simulink model "main_pipeline"  (R2021a)
settings: Solver=FixedStepDiscrete  StartTime=0.0  StopTime=0  RelTol=1e-3
undefined symbols (not defined in the file): gray, Rec, SDTV, strel
libraries: visiontextngfix x9, visionmorphops x7, visionstatistics x3, visionconversions x2, visionsources x1
settings Model: Creator=leonardoaraujo  LastModifiedBy=leonardoaraujo

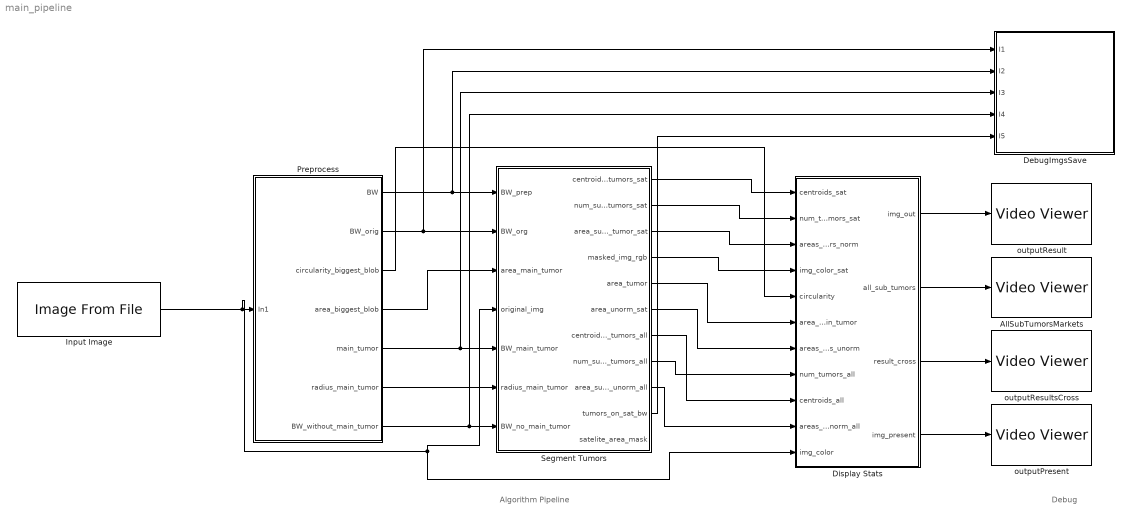
== system main_pipeline ==
  note: Algorithm Pipeline
  note: Debug
  AllSubTumorsMarkets : VideoViewer  colormapValue=gray(256)  FigPos=[659 848 678 632]
  DebugImgsSave : MATLAB Function  TreatAsAtomicUnit=on
  Display Stats : Subsystem
  Input Image : visionsources/Image From File  Tag=vipblks_nd  FileName=/Users/leonardoaraujo/Desktop/Cher Experiment/C6R_OV_BiggerBrain.jpg  Ts=inf  imagePorts=One multidimensional signal  OutPortLabels=R|G|B  ImageDataType=Inherit from input image  sdImageDataType=uint(8)  Signed=on  WordLength=16  FractionLengthMode=User-defined  FractionLength=15
  Preprocess : Subsystem  mask{open_1=8, erode_1=2, close_1=10}
      mask prompts: open_1 "Open Blobs"; erode_1 "Pre-clean"; close_1 "Close Main tumor"
  Segment Tumors : Subsystem  mask{erode_1=2, sat_area=150}
      mask prompts: erode_1 "Filter Small Artifacts"; sat_area "Satelite Area"
  outputPresent : VideoViewer  colormapValue=gray(256)  FigPos=[1 849 1440 721]
  outputResult : VideoViewer  colormapValue=gray(256)  FigPos=[180 848 678 632]
  outputResultsCross : VideoViewer  colormapValue=gray(256)  FigPos=[415 815 678 632]
  wires:
  Input Image/1 -> Segment Tumors/4(original_img), Display Stats/11(img_color), Preprocess/1(In1)
  Preprocess/1(BW) -> DebugImgsSave/2(I2), Segment Tumors/1(BW_prep)
  Preprocess/2(BW_orig) -> DebugImgsSave/1(I1), Segment Tumors/2(BW_org)
  Segment Tumors/1(centroid_sub_tumors_sat) -> Display Stats/1(centroids_sat)
  Segment Tumors/2(num_sub_tumors_sat) -> Display Stats/2(num_tumors_sat)
  Segment Tumors/3(area_sub_tumor_sat) -> Display Stats/3(areas_sub_tumors_norm)
  Preprocess/3(circularity_biggest_blob) -> Display Stats/5(circularity)
  Preprocess/4(area_biggest_blob) -> Segment Tumors/3(area_main_tumor)
  Segment Tumors/4(masked_img_rgb) -> Display Stats/4(img_color_sat)
  Segment Tumors/5(area_tumor) -> Display Stats/6(area_main_tumor)
  Segment Tumors/10(tumors_on_sat_bw) -> DebugImgsSave/5(I5)
  Segment Tumors/6(area_unorm_sat) -> Display Stats/7(areas_sub_tumors_unorm)
  Display Stats/1(img_out) -> outputResult/1
  Segment Tumors/8(num_sub_tumors_all) -> Display Stats/8(num_tumors_all)
  Segment Tumors/7(centroid_sub_tumors_all) -> Display Stats/9(centroids_all)
  Segment Tumors/9(area_sub_tumors_unorm_all) -> Display Stats/10(areas_sub_tumors_unorm_all)
  Display Stats/2(all_sub_tumors) -> AllSubTumorsMarkets/1
  Preprocess/5(main_tumor) -> DebugImgsSave/3(I3), Segment Tumors/5(BW_main_tumor)
  Preprocess/6(radius_main_tumor) -> Segment Tumors/6(radius_main_tumor)
  Preprocess/7(BW_without_main_tumor) -> DebugImgsSave/4(I4), Segment Tumors/7(BW_no_main_tumor)
  Display Stats/3(result_cross) -> outputResultsCross/1
  Display Stats/4(img_present) -> outputPresent/1

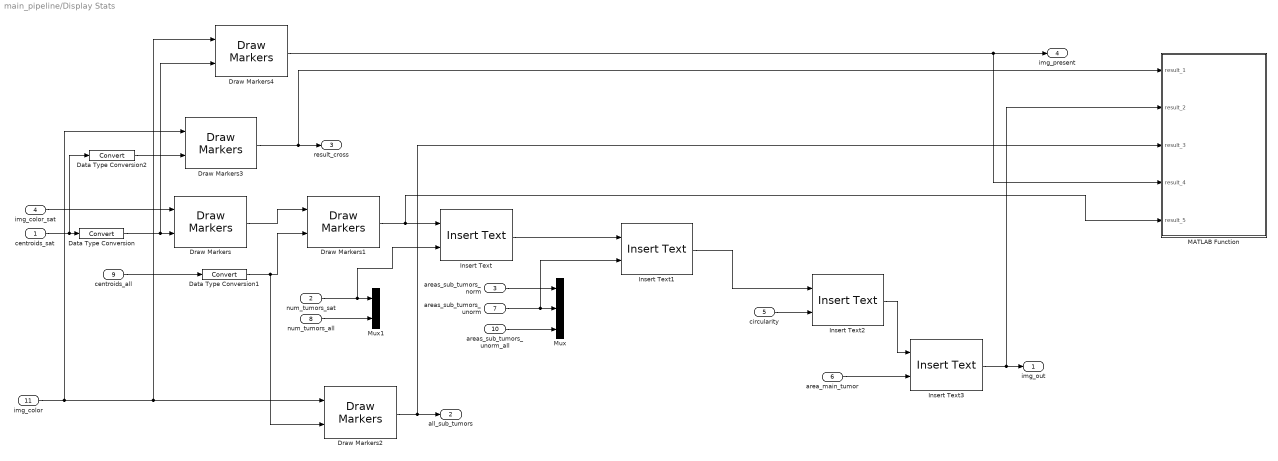
== system main_pipeline/Display Stats ==
  centroids_sat : Inport
  num_tumors_sat : Inport  Port=2
  areas_sub_tumors_norm : Inport  Port=3
  img_color_sat : Inport  Port=4
  circularity : Inport  Port=5
  area_main_tumor : Inport  Port=6
  areas_sub_tumors_unorm : Inport  Port=7
  num_tumors_all : Inport  Port=8
  centroids_all : Inport  Port=9
  areas_sub_tumors_unorm_all : Inport  Port=10
  img_color : Inport  Port=11
  Data Type Conversion : DataTypeConversion
  Data Type Conversion1 : DataTypeConversion
  Data Type Conversion2 : DataTypeConversion
  Draw Markers : visiontextngfix/Draw Markers  shape=Circle  size=30  fill=on  fillClrSource=Specify via dialog  display=User-specified value  intensity=200  color=[200 0 0]  opacity=0.6  viewport=Entire image  antialiasing=off  inType=Obsolete  imagePorts=One multidimensional signal  roundingMode=Floor  overflowMode=off  memoryMode=Specify word length  memoryWordLength=16  memoryFracLength=15  prodOutputMode=Binary point scaling  prodOutputWordLength=32  prodOutputFracLength=14
      settings: SourceProductBaseCode=VP
  Draw Markers1 : visiontextngfix/Draw Markers  shape=Circle  size=10  fill=on  fillClrSource=Specify via dialog  display=User-specified value  intensity=200  color=[0 0 200]  opacity=0.3  viewport=Entire image  antialiasing=off  inType=Obsolete  imagePorts=One multidimensional signal  roundingMode=Floor  overflowMode=off  memoryMode=Specify word length  memoryWordLength=16  memoryFracLength=15  prodOutputMode=Binary point scaling  prodOutputWordLength=32  prodOutputFracLength=14
      settings: SourceProductBaseCode=VP
  Draw Markers2 : visiontextngfix/Draw Markers  shape=Circle  size=10  fill=on  fillClrSource=Specify via dialog  display=User-specified value  intensity=200  color=[0 0 200]  opacity=0.3  viewport=Entire image  antialiasing=off  inType=Obsolete  imagePorts=One multidimensional signal  roundingMode=Floor  overflowMode=off  memoryMode=Specify word length  memoryWordLength=16  memoryFracLength=15  prodOutputMode=Binary point scaling  prodOutputWordLength=32  prodOutputFracLength=14
      settings: SourceProductBaseCode=VP
  Draw Markers3 : visiontextngfix/Draw Markers  shape=Plus  size=30  fill=on  fillClrSource=Specify via dialog  display=User-specified value  intensity=200  color=[200 0 0]  opacity=0.6  viewport=Entire image  antialiasing=off  inType=Obsolete  imagePorts=One multidimensional signal  roundingMode=Floor  overflowMode=off  memoryMode=Specify word length  memoryWordLength=16  memoryFracLength=15  prodOutputMode=Binary point scaling  prodOutputWordLength=32  prodOutputFracLength=14
      settings: SourceProductBaseCode=VP
  Draw Markers4 : visiontextngfix/Draw Markers  shape=Circle  size=30  fill=on  fillClrSource=Specify via dialog  display=User-specified value  intensity=200  color=[200 0 0]  opacity=0.6  viewport=Entire image  antialiasing=off  inType=Obsolete  imagePorts=One multidimensional signal  roundingMode=Floor  overflowMode=off  memoryMode=Specify word length  memoryWordLength=16  memoryFracLength=15  prodOutputMode=Binary point scaling  prodOutputWordLength=32  prodOutputFracLength=14
      settings: SourceProductBaseCode=VP
  Insert Text : visiontextngfix/Insert Text  inputType=Obsolete  theText='#Satellite Lesion: %2d'  getTextLocFrom=Specify via dialog  textLoc=[1 1]  getTextColorFrom=Specify via dialog  textColor=[0 255 0]  getTextIntensityFrom=Specify via dialog  textIntensity=100  getTextOpacityFrom=Specify via dialog  textOpacity=1.0  dummyVar2=0  dummyVar3=0  dummyVar4=0  imagePorts=One multidimensional signal  isInputTransposed=off  fontFace=LucidaSansRegular  dummyVar1=0  blockFontSize=25  antiAliased=on
      settings: SourceProductBaseCode=VP
  Insert Text1 : visiontextngfix/Insert Text  inputType=Obsolete  theText='Satellite Lesion Total Area: %2f'  getTextLocFrom=Specify via dialog  textLoc=[1 50]  getTextColorFrom=Specify via dialog  textColor=[0 255 0]  getTextIntensityFrom=Specify via dialog  textIntensity=100  getTextOpacityFrom=Specify via dialog  textOpacity=1.0  dummyVar2=0  dummyVar3=0  dummyVar4=0  imagePorts=One multidimensional signal  isInputTransposed=off  fontFace=LucidaSansRegular  dummyVar1=0  blockFontSize=25  antiAliased=on
      settings: SourceProductBaseCode=VP
  Insert Text2 : visiontextngfix/Insert Text  inputType=Obsolete  theText='Surface Irregularity: %2f'  getTextLocFrom=Specify via dialog  textLoc=[1 100]  getTextColorFrom=Specify via dialog  textColor=[0 255 0]  getTextIntensityFrom=Specify via dialog  textIntensity=100  getTextOpacityFrom=Specify via dialog  textOpacity=1.0  dummyVar2=0  dummyVar3=0  dummyVar4=0  imagePorts=One multidimensional signal  isInputTransposed=off  fontFace=LucidaSansRegular  dummyVar1=0  blockFontSize=25  antiAliased=on
      settings: SourceProductBaseCode=VP
  Insert Text3 : visiontextngfix/Insert Text  inputType=Obsolete  theText='Main tumor Size: %d'  getTextLocFrom=Specify via dialog  textLoc=[1 150]  getTextColorFrom=Specify via dialog  textColor=[0 255 0]  getTextIntensityFrom=Specify via dialog  textIntensity=100  getTextOpacityFrom=Specify via dialog  textOpacity=1.0  dummyVar2=0  dummyVar3=0  dummyVar4=0  imagePorts=One multidimensional signal  isInputTransposed=off  fontFace=LucidaSansRegular  dummyVar1=0  blockFontSize=25  antiAliased=on
      settings: SourceProductBaseCode=VP
  MATLAB Function : MATLAB Function  TreatAsAtomicUnit=on
  Mux : Mux  Inputs=3
  Mux1 : Mux  Inputs=2
  img_out : Outport
  all_sub_tumors : Outport  Port=2
  result_cross : Outport  Port=3
  img_present : Outport  Port=4
  wires:
  Data Type Conversion/1 -> Draw Markers4/2, Draw Markers/2
  centroids_sat/1 -> Data Type Conversion2/1, Data Type Conversion/1
  img_color_sat/1 -> Draw Markers/1
  Insert Text/1 -> Insert Text1/1
  Insert Text1/1 -> Insert Text2/1
  circularity/1 -> Insert Text2/2
  Insert Text2/1 -> Insert Text3/1
  Insert Text3/1 -> MATLAB Function/2(result_2), img_out/1
  area_main_tumor/1 -> Insert Text3/2
  areas_sub_tumors_norm/1 -> Mux/1
  areas_sub_tumors_unorm/1 -> Insert Text1/2, Mux/2
  num_tumors_sat/1 -> Insert Text/2, Mux1/1
  Draw Markers/1 -> Draw Markers1/1
  Draw Markers1/1 -> MATLAB Function/5(result_5), Insert Text/1
  centroids_all/1 -> Data Type Conversion1/1
  Data Type Conversion1/1 -> Draw Markers2/2, Draw Markers1/2
  areas_sub_tumors_unorm_all/1 -> Mux/3
  Draw Markers2/1 -> MATLAB Function/3(result_3), all_sub_tumors/1
  img_color/1 -> Draw Markers2/1, Draw Markers4/1, Draw Markers3/1
  Data Type Conversion2/1 -> Draw Markers3/2
  Draw Markers3/1 -> MATLAB Function/1(result_1), result_cross/1
  Draw Markers4/1 -> img_present/1, MATLAB Function/4(result_4)
  num_tumors_all/1 -> Mux1/2

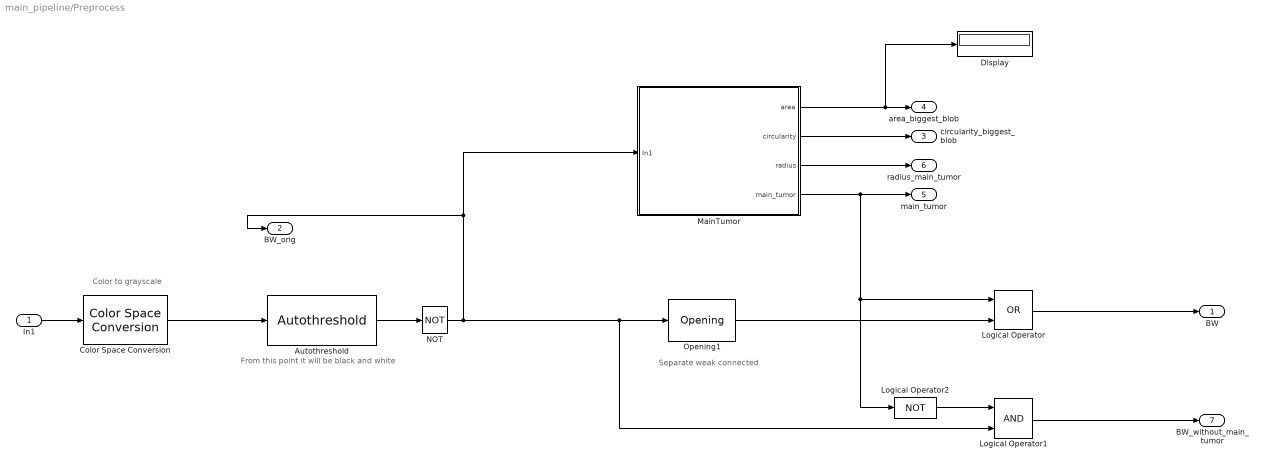
== system main_pipeline/Preprocess ==
  note: From this point it will be black and white
  note: Color to grayscale
  note: Separate weak connected
  In1 : Inport
  Autothreshold : visionconversions/Autothreshold  operator=>  threshOut=off  effMetricOut=off  userDefinedRange=off  umin=0  umax=255  outOfRngOpt=Ignore  scaleThreshold=off  scaleFactor=1  roundingMode=Floor  overflowMode=off  P1Mode=Specify word length  P1WordLength=32  P1FracLength=30  P2Mode=Specify word length  P2WordLength=32  P2FracLength=22  P3Mode=Specify word length  P3WordLength=32  P3FracLength=14  P4Mode=Binary point scaling  P4WordLength=32  P4FracLength=15  Q1Mode=Specify word length  Q1WordLength=32  Q1FracLength=16  EMMode=Specify word length  EMWordLength=16  EMFracLength=14
      settings: SourceProductBaseCode=VP
  Color Space Conversion : visionconversions/Color Space  Conversion  conversion=Obsolete  conversionActive=R'G'B' to intensity  wp_str=D65  rec=Rec. 601 (SDTV)  sys=1125/60/2:1  imagePorts=One multidimensional signal
  Display : Display
  Logical Operator : Logic  Operator=OR  AllPortsSameDT=off  OutDataTypeStr=boolean
  Logical Operator1 : Logic  AllPortsSameDT=off  OutDataTypeStr=boolean
  Logical Operator2 : Logic  Operator=NOT  AllPortsSameDT=off  OutDataTypeStr=boolean
  MainTumor : Subsystem
  NOT : Logic  Operator=NOT  IconShape=distinctive  AllPortsSameDT=off  OutDataTypeStr=boolean
  Opening1 : visionmorphops/Opening  nhoodsrc=Specify via dialog  strel=strel('disk',open_1)
      settings: SourceProductBaseCode=VP
  BW : Outport
  BW_orig : Outport  Port=2
  circularity_biggest_blob : Outport  Port=3
  area_biggest_blob : Outport  Port=4
  main_tumor : Outport  Port=5
  radius_main_tumor : Outport  Port=6
  BW_without_main_tumor : Outport  Port=7
  wires:
  Autothreshold/1 -> NOT/1
  In1/1 -> Color Space Conversion/1
  Opening1/1 -> Logical Operator/2
  Color Space Conversion/1 -> Autothreshold/1
  MainTumor/2(circularity) -> circularity_biggest_blob/1
  MainTumor/3(radius) -> radius_main_tumor/1
  MainTumor/4(main_tumor) -> Logical Operator2/1, Logical Operator/1, main_tumor/1
  MainTumor/1(area) -> Display/1, area_biggest_blob/1
  Logical Operator/1 -> BW/1
  Logical Operator2/1 -> Logical Operator1/1
  Logical Operator1/1 -> BW_without_main_tumor/1
  NOT/1 -> Logical Operator1/2, Opening1/1, MainTumor/1(In1), BW_orig/1

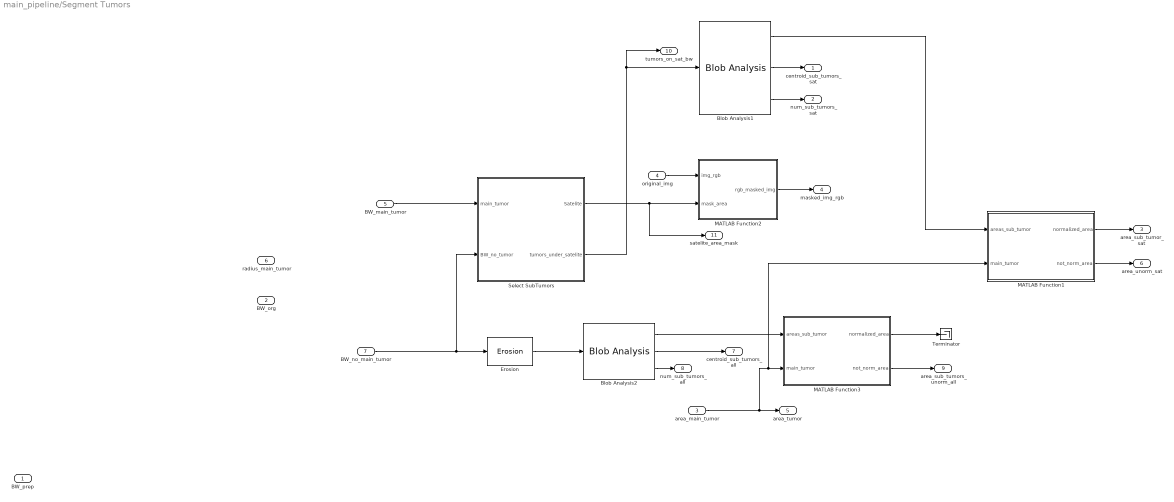
== system main_pipeline/Segment Tumors ==
  BW_prep : Inport
  BW_org : Inport  Port=2
  area_main_tumor : Inport  Port=3
  original_img : Inport  Port=4
  BW_main_tumor : Inport  Port=5
  radius_main_tumor : Inport  Port=6
  BW_no_main_tumor : Inport  Port=7
  Blob Analysis1 : visionstatistics/Blob Analysis  Tag=vipblks_row_conv  area=on  centroid=on  bBox=off  majorAxis=off  minorAxis=off  angle=off  eccentricity=off  equivDiameterSq=off  extent=off  perimeter=off  outDT=double  conn=8  isLabel=off  maxBlobs=500  warnIfNumBlobsExceeded=on  isCount=on  useMinArea=off  minArea=0  useMaxArea=off  maxArea=intmax('uint32')  excludeBorderBlob=on  isOutVarDim=off  isFill=on  fillValues=-1  roundingMode=Floor  overflowMode=off  prodOutputMode=Binary point scaling  prodOutputWordLength=32  prodOutputFracLength=16  accumMode=Binary point scaling  accumWordLength=32  accumFracLength=0  outputMode=Binary point scaling  outputWordLength=32  outputFracLength=16  firstCoeffMode=Binary point scaling  firstCoeffWordLength=16  firstCoeffFracLength=14  secondCoeffMode=Binary point scaling  secondCoeffWordLength=32  secondCoeffFracLength=16
  Blob Analysis2 : visionstatistics/Blob Analysis  Tag=vipblks_row_conv  area=on  centroid=on  bBox=off  majorAxis=off  minorAxis=off  angle=off  eccentricity=off  equivDiameterSq=off  extent=off  perimeter=off  outDT=double  conn=8  isLabel=off  maxBlobs=500  warnIfNumBlobsExceeded=on  isCount=on  useMinArea=off  minArea=0  useMaxArea=off  maxArea=intmax('uint32')  excludeBorderBlob=on  isOutVarDim=off  isFill=on  fillValues=-1  roundingMode=Floor  overflowMode=off  prodOutputMode=Binary point scaling  prodOutputWordLength=32  prodOutputFracLength=16  accumMode=Binary point scaling  accumWordLength=32  accumFracLength=0  outputMode=Binary point scaling  outputWordLength=32  outputFracLength=16  firstCoeffMode=Binary point scaling  firstCoeffWordLength=16  firstCoeffFracLength=14  secondCoeffMode=Binary point scaling  secondCoeffWordLength=32  secondCoeffFracLength=16
  Erosion : visionmorphops/Erosion  nhoodsrc=Specify via dialog  strel=strel('disk',erode_1)
      settings: SourceProductBaseCode=VP
  MATLAB Function1 : MATLAB Function  TreatAsAtomicUnit=on
  MATLAB Function2 : MATLAB Function  TreatAsAtomicUnit=on
  MATLAB Function3 : MATLAB Function  TreatAsAtomicUnit=on
  Select SubTumors : Subsystem
  Terminator : Terminator
  centroid_sub_tumors_sat : Outport
  num_sub_tumors_sat : Outport  Port=2
  area_sub_tumor_sat : Outport  Port=3
  masked_img_rgb : Outport  Port=4
  area_tumor : Outport  Port=5
  area_unorm_sat : Outport  Port=6
  centroid_sub_tumors_all : Outport  Port=7
  num_sub_tumors_all : Outport  Port=8
  area_sub_tumors_unorm_all : Outport  Port=9
  tumors_on_sat_bw : Outport  Port=10
  satelite_area_mask : Outport  Port=11
  wires:
  Blob Analysis2/2 -> centroid_sub_tumors_all/1
  Blob Analysis2/1 -> MATLAB Function3/1(areas_sub_tumor)
  Blob Analysis2/3 -> num_sub_tumors_all/1
  MATLAB Function3/1(normalized_area) -> Terminator/1
  MATLAB Function3/2(not_norm_area) -> area_sub_tumors_unorm_all/1
  area_main_tumor/1 -> MATLAB Function1/2(main_tumor), MATLAB Function3/2(main_tumor), area_tumor/1
  BW_no_main_tumor/1 -> Select SubTumors/2(BW_no_tumor), Erosion/1
  BW_main_tumor/1 -> Select SubTumors/1(main_tumor)
  MATLAB Function2/1(rgb_masked_img) -> masked_img_rgb/1
  original_img/1 -> MATLAB Function2/1(img_rgb)
  Select SubTumors/1(Satelite) -> satelite_area_mask/1, MATLAB Function2/2(mask_area)
  Select SubTumors/2(tumors_under_satelite) -> tumors_on_sat_bw/1, Blob Analysis1/1
  Blob Analysis1/1 -> MATLAB Function1/1(areas_sub_tumor)
  Blob Analysis1/2 -> centroid_sub_tumors_sat/1
  Blob Analysis1/3 -> num_sub_tumors_sat/1
  MATLAB Function1/2(not_norm_area) -> area_unorm_sat/1
  MATLAB Function1/1(normalized_area) -> area_sub_tumor_sat/1
  Erosion/1 -> Blob Analysis2/1

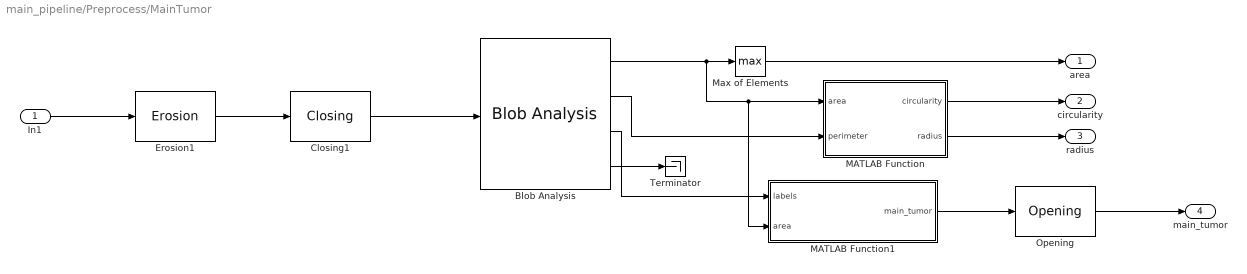
== system main_pipeline/Preprocess/MainTumor ==
  In1 : Inport
  Blob Analysis : visionstatistics/Blob Analysis  Tag=vipblks_row_conv  area=on  centroid=off  bBox=off  majorAxis=off  minorAxis=off  angle=off  eccentricity=off  equivDiameterSq=off  extent=off  perimeter=on  outDT=double  conn=8  isLabel=on  maxBlobs=50  warnIfNumBlobsExceeded=on  isCount=on  useMinArea=on  minArea=200  useMaxArea=off  maxArea=intmax('uint32')  excludeBorderBlob=on  isOutVarDim=off  isFill=on  fillValues=-1  roundingMode=Floor  overflowMode=off  prodOutputMode=Binary point scaling  prodOutputWordLength=32  prodOutputFracLength=16  accumMode=Binary point scaling  accumWordLength=32  accumFracLength=0  outputMode=Binary point scaling  outputWordLength=32  outputFracLength=16  firstCoeffMode=Binary point scaling  firstCoeffWordLength=16  firstCoeffFracLength=14  secondCoeffMode=Binary point scaling  secondCoeffWordLength=32  secondCoeffFracLength=16
  Closing1 : visionmorphops/Closing  nhoodsrc=Specify via dialog  strel=strel('disk',close_1)
      settings: SourceProductBaseCode=VP
  Erosion1 : visionmorphops/Erosion  nhoodsrc=Specify via dialog  strel=strel('disk',erode_1)
      settings: SourceProductBaseCode=VP
  MATLAB Function : MATLAB Function  TreatAsAtomicUnit=on
  MATLAB Function1 : MATLAB Function  TreatAsAtomicUnit=on
  Max of Elements : MinMax  Function=max
  Opening : visionmorphops/Opening  nhoodsrc=Specify via dialog  strel=strel('disk',30)
      settings: SourceProductBaseCode=VP
  Terminator : Terminator
  area : Outport
  circularity : Outport  Port=2
  radius : Outport  Port=3
  main_tumor : Outport  Port=4
  wires:
  Blob Analysis/4 -> Terminator/1
  In1/1 -> Erosion1/1
  Blob Analysis/3 -> MATLAB Function1/1(labels)
  Max of Elements/1 -> area/1
  Blob Analysis/1 -> MATLAB Function/1(area), MATLAB Function1/2(area), Max of Elements/1
  MATLAB Function/2(radius) -> radius/1
  MATLAB Function/1(circularity) -> circularity/1
  Blob Analysis/2 -> MATLAB Function/2(perimeter)
  Erosion1/1 -> Closing1/1
  Closing1/1 -> Blob Analysis/1
  Opening/1 -> main_tumor/1
  MATLAB Function1/1(main_tumor) -> Opening/1

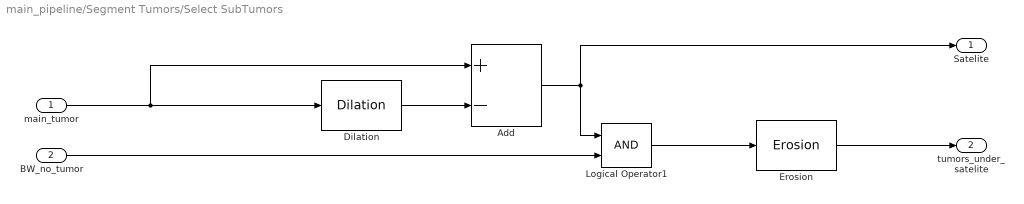
== system main_pipeline/Segment Tumors/Select SubTumors ==
  main_tumor : Inport
  BW_no_tumor : Inport  Port=2
  Add : Sum  Inputs=+-
  Dilation : visionmorphops/Dilation  nhoodsrc=Specify via dialog  strel=strel('disk',sat_area)
      settings: SourceProductBaseCode=VP
  Erosion : visionmorphops/Erosion  nhoodsrc=Specify via dialog  strel=strel('disk',erode_1)
      settings: SourceProductBaseCode=VP
  Logical Operator1 : Logic  AllPortsSameDT=off  OutDataTypeStr=boolean
  Satelite : Outport
  tumors_under_satelite : Outport  Port=2
  wires:
  Dilation/1 -> Add/2
  BW_no_tumor/1 -> Logical Operator1/2
  Add/1 -> Satelite/1, Logical Operator1/1
  main_tumor/1 -> Dilation/1, Add/1
  Logical Operator1/1 -> Erosion/1
  Erosion/1 -> tumors_under_satelite/1

== matlab function main_pipeline/Segment Tumors/MATLAB Function1 ==
  data: areas_sub_tumor input; normalized_area output; main_tumor input; not_norm_area output
function [normalized_area, not_norm_area] = stats_sub_tumor(areas_sub_tumor, main_tumor)

normalized_area = sum(areas_sub_tumor) / double(main_tumor);
not_norm_area = sum(areas_sub_tumor);

== matlab function main_pipeline/Display Stats/MATLAB Function ==
  data: result_1 input; result_2 input; result_3 input; result_4 input; result_5 input
function save_imgs(result_1, result_2, result_3, result_4, result_5)
% Declare imwrite as extrinsic to avoid code generation
coder.extrinsic('imwrite');
imwrite(result_1, './result_cross.tif');
imwrite(result_2, './result_with_stats.tif');
imwrite(result_3, './result_all_tumors.tif');
imwrite(result_4, './beautiful.tif');
imwrite(result_5, './pink_no_text.tif');

== matlab function main_pipeline/Segment Tumors/MATLAB Function2 ==
  data: img_rgb input; rgb_masked_img output; mask_area input
function rgb_masked_img = mask_color_image(img_rgb, mask_area)

% Mask the original image with the mask
rgb_masked_img = img_rgb;
for channels = 1:3
    rgb_masked_img(:,:,2) = img_rgb(:,:,channels) .* mask_area;
end

== matlab function main_pipeline/Preprocess/MainTumor/MATLAB Function ==
  data: area input; circularity output; perimeter input; radius output
function [circularity, radius] = get_circularity(area, perimeter)
% References
% https://uk.mathworks.com/matlabcentral/answers/108115-determine-shape-smoothness-roughness
[biggest_area, idx_biggest] = max(area);
perimeter_biggest = perimeter(idx_biggest);
% A perfect circle will be 1 (This is normalized)
circularity = (perimeter_biggest^2) / (4*pi*double(biggest_area));
radius = perimeter(idx_biggest) / (2*pi);

== matlab function main_pipeline/Segment Tumors/MATLAB Function3 ==
  data: areas_sub_tumor input; normalized_area output; main_tumor input; not_norm_area output
function [normalized_area, not_norm_area] = stats_sub_tumor(areas_sub_tumor, main_tumor)

normalized_area = sum(areas_sub_tumor) / double(main_tumor);
not_norm_area = sum(areas_sub_tumor);

== matlab function main_pipeline/Preprocess/MainTumor/MATLAB Function1 ==
  data: labels input; main_tumor output; area input
function main_tumor = select_main_tumor(labels, area)
[~, idx_biggest] = max(area);
main_tumor = logical((labels == idx_biggest));
% Choose a big close to garantee that the main tumor is closed
morph_element = strel('disk', 10);
main_tumor = logical(~imerode(~main_tumor, morph_element));

== matlab function main_pipeline/DebugImgsSave ==
  data: I1 input; I2 input; I3 input; I4 input; I5 input
function save_imgs_debug(I1, I2, I3, I4, I5)
% Declare imwrite as extrinsic to avoid code generation
coder.extrinsic('imwrite');
imwrite(I1, './BW_original.tif');
imwrite(I2, './BW_prepared.tif');
imwrite(I3, './main_tumor.tif');
imwrite(I4, './BW_no_tumor.tif');
imwrite(I5, './tumors_on_sat.tif');
